simulink model "SignalProcessing2"  (R2016b)
settings: Solver=VariableStepAuto  StartTime=0.0  StopTime=5  RelTol=1e-3
libraries: dspstat3 x4, dspsigops x3, simulink x1, dspfdesign x1
settings Model: Creator=Ege  LastModifiedBy=Ege

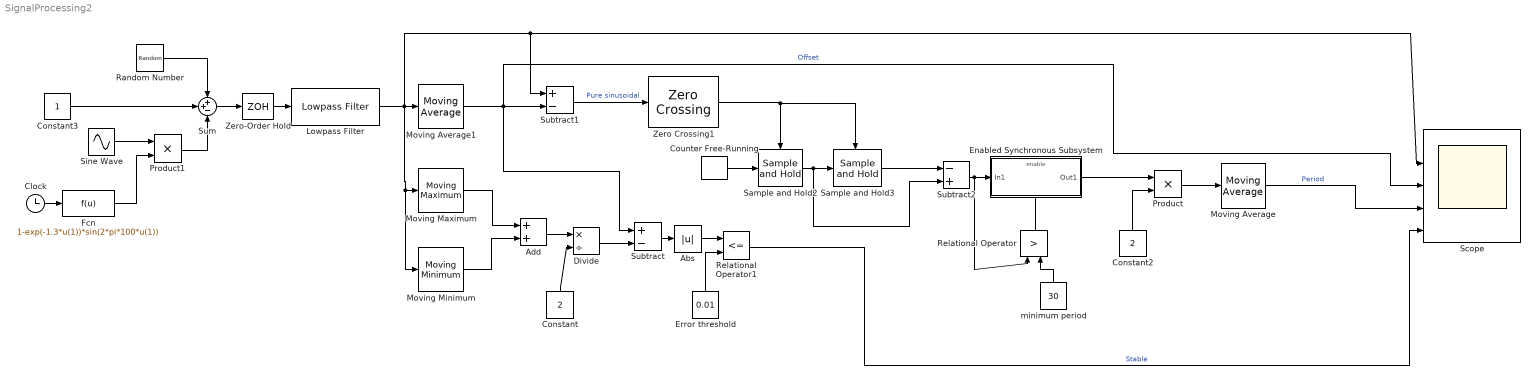
== system SignalProcessing2 ==
  Abs : Abs
  Add : Sum
  Clock : Clock
  Constant : Constant  Value=2
  Constant2 : Constant  Value=2
  Constant3 : Constant
  Counter Free-Running : simulink/Sources/Counter Free-Running  NumBits=16  tsamp=-1
  Divide : Product  Inputs=*/
  Enabled Synchronous Subsystem : Subsystem  TreatAsAtomicUnit=on
  Error threshold : Constant  Value=0.01
  Fcn : Fcn  Expr=1-exp(-1.3*u(1))*sin(2*pi*100*u(1))
  Lowpass Filter : dspfdesign/Lowpass Filter  FilterType=FIR  DesignForMinimumOrder=on  FilterOrder=50  PassbandFrequency=1e3  StopbandFrequency=2e3  PassbandRipple=0.1  StopbandAttenuation=80  InheritSampleRate=on  SampleRate=44100  SimulateUsing=Interpreted execution  roundingMode=Floor  coeffsDataTypeStr=fixdt(1,16)
  Moving Average : dspstat3/Moving Average  Method=Sliding window  SpecifyWindowLength=on  WindowLength=10000  ForgettingFactor=0.1  SimulateUsing=Code generation
  Moving Average1 : dspstat3/Moving Average  Method=Sliding window  SpecifyWindowLength=on  WindowLength=10000  ForgettingFactor=0.1  SimulateUsing=Code generation
  Moving Maximum : dspstat3/Moving Maximum  SpecifyWindowLength=on  WindowLength=10000  SimulateUsing=Code generation
  Moving Minimum : dspstat3/Moving Minimum  SpecifyWindowLength=on  WindowLength=10000  SimulateUsing=Code generation
  Product : Product
  Product1 : Product
  Random Number : RandomNumber  Variance=0.01  SampleTime=0.0001
  Relational Operator : RelationalOperator  Operator=>  OutDataTypeStr=boolean  RndMeth=Nearest
  Relational Operator1 : RelationalOperator  Operator=<=  OutDataTypeStr=boolean  RndMeth=Simplest
  Sample and Hold2 : dspsigops/Sample and Hold  trig=Rising edge  initCond=0  latchinput=on
  Sample and Hold3 : dspsigops/Sample and Hold  trig=Rising edge  initCond=0  latchinput=on
  Scope : Scope  NumInputPorts=5
  Sine Wave : Sin  Frequency=100*2*pi  SampleTime=0
  Subtract : Sum  Inputs=+-
  Subtract1 : Sum  Inputs=+-
  Subtract2 : Sum  Inputs=-+  AccumDataTypeStr=fixdt(0,16,0)
  Sum : Sum  Inputs=++-
  Zero Crossing1 : dspsigops/Zero Crossing  InputProcessing=Columns as channels (frame based)
  Zero-Order Hold : ZeroOrderHold  SampleTime=0.0001
  minimum period : Constant  Value=30
  wires:
  Clock/1 -> Fcn/1
  Zero-Order Hold/1 -> Lowpass Filter/1
  Random Number/1 -> Sum/1
  Moving Average1/1 -> Scope/3, Subtract/1, Subtract1/2  "Offset"
  Subtract1/1 -> Zero Crossing1/1  "Pure sinusoidal"
  Sample and Hold2/1 -> Subtract2/2, Sample and Hold3/1
  Counter Free-Running/1 -> Sample and Hold2/1
  Zero Crossing1/1 -> Sample and Hold3/Trigger, Sample and Hold2/Trigger
  Sample and Hold3/1 -> Subtract2/1
  Constant2/1 -> Product/2
  Product/1 -> Moving Average/1
  Subtract2/1 -> Enabled Synchronous Subsystem/1(In1), Relational Operator/1
  minimum period/1 -> Relational Operator/2
  Relational Operator/1 -> Enabled Synchronous Subsystem/Enable
  Enabled Synchronous Subsystem/1(Out1) -> Product/1
  Sum/1 -> Zero-Order Hold/1
  Lowpass Filter/1 -> Moving Minimum/1, Moving Maximum/1, Moving Average1/1, Scope/2, Subtract1/1
  Moving Maximum/1 -> Add/1
  Moving Minimum/1 -> Add/2
  Add/1 -> Divide/1
  Constant/1 -> Divide/2
  Divide/1 -> Subtract/2
  Subtract/1 -> Abs/1
  Abs/1 -> Relational Operator1/1
  Error threshold/1 -> Relational Operator1/2
  Relational Operator1/1 -> Scope/5  "Stable"
  Moving Average/1 -> Scope/4  "Period"
  Sine Wave/1 -> Product1/1
  Fcn/1 -> Product1/2
  Product1/1 -> Sum/3
  Constant3/1 -> Sum/2

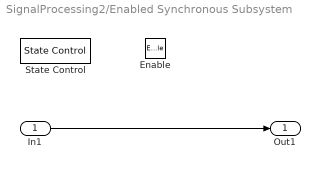
== system SignalProcessing2/Enabled Synchronous Subsystem ==
  In1 : Inport
  Enable : EnablePort
  State Control : StateControl
  Out1 : Outport
  wires:
  In1/1 -> Out1/1
